simulink model "c_station_v3"  (R2019a)
settings: Solver=VariableStepAuto  StartTime=0.0  StopTime=604800  MaxStep=3600  RelTol=1e-3  AbsTol=1e-3  EnableMultiTasking=on
StopFcn:
  | displayGasParameters(gasPressures);
values from neighbouring files (symbols this model uses):
  conf = gasConfig()    [gas_v1.m]
  valveControlFlag = "on"    [gas_v1.m]
undefined symbols (not defined in the file or in its folder): lineParm, loadParm, valveParm
libraries: gasLibrary x25, fl_lib x19, nesl_utility x11, SimscapeFluids_lib x1
(part 3 of 3)

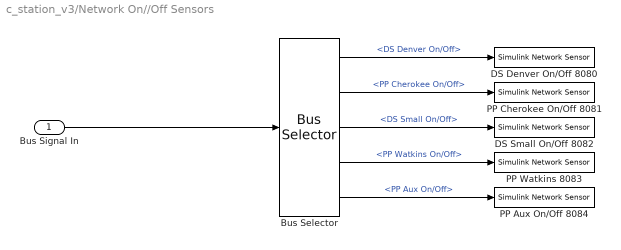
== system c_station_v3/Network On//Off Sensors ==
  Bus Signal In : Inport
  Bus Selector : BusSelector  OutputSignals=DS Denver On/Off,PP Cherokee On/Off,DS Small On/Off,PP Watkins On/Off,PP Aux On/Off
  DS Denver On/Off 8080 : gasLibrary/Simulink Network Sensor  Port=8080
  DS Small On/Off 8082 : gasLibrary/Simulink Network Sensor  Port=8082
  PP Aux On/Off 8084 : gasLibrary/Simulink Network Sensor  Port=8084
  PP Cherokee On/Off 8081 : gasLibrary/Simulink Network Sensor  Port=8081
  PP Watkins 8083 : gasLibrary/Simulink Network Sensor  Port=8083
  wires:
  Bus Selector/1 -> DS Denver On/Off 8080/1  "<DS Denver On/Off>"
  Bus Signal In/1 -> Bus Selector/1
  Bus Selector/2 -> PP Cherokee On/Off 8081/1  "<PP Cherokee On/Off>"
  Bus Selector/4 -> PP Watkins 8083/1  "<PP Watkins On/Off>"
  Bus Selector/5 -> PP Aux On/Off 8084/1  "<PP Aux On/Off>"
  Bus Selector/3 -> DS Small On/Off 8082/1  "<DS Small On/Off>"

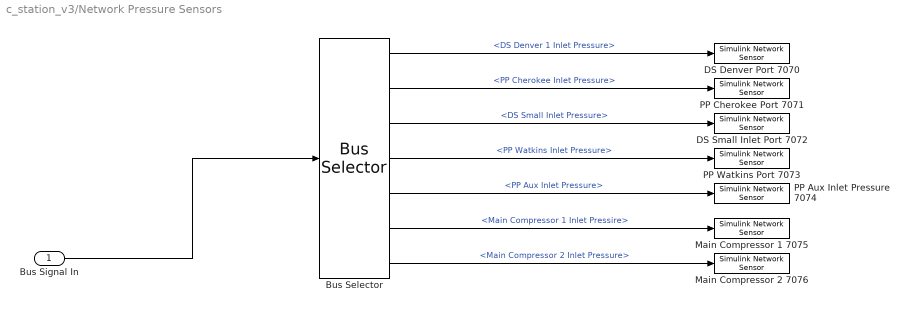
== system c_station_v3/Network Pressure Sensors ==
  Bus Signal In : Inport
  Bus Selector : BusSelector  OutputSignals=DS Denver 1 Inlet Pressure,PP Cherokee Inlet Pressure,DS Small Inlet Pressure,PP Watkins Inlet Pressure,PP Aux Inlet Pressure,Main Compressor 1 Inlet Pressire,Main Compressor 2 Inlet Pressure
  DS Denver Port 7070 : gasLibrary/Simulink Network Sensor  Port=7070
  DS Small Inlet Port 7072 : gasLibrary/Simulink Network Sensor  Port=7072
  Main Compressor 1 7075 : gasLibrary/Simulink Network Sensor  Port=7075
  Main Compressor 2 7076 : gasLibrary/Simulink Network Sensor  Port=7076
  PP Aux Inlet Pressure 7074 : gasLibrary/Simulink Network Sensor  Port=7074
  PP Cherokee Port 7071 : gasLibrary/Simulink Network Sensor  Port=7071
  PP Watkins Port 7073 : gasLibrary/Simulink Network Sensor  Port=7073
  wires:
  Bus Selector/4 -> PP Watkins Port 7073/1  "<PP Watkins Inlet Pressure>"
  Bus Signal In/1 -> Bus Selector/1
  Bus Selector/2 -> PP Cherokee Port 7071/1  "<PP Cherokee Inlet Pressure>"
  Bus Selector/3 -> DS Small Inlet Port 7072/1  "<DS Small Inlet Pressure>"
  Bus Selector/1 -> DS Denver Port 7070/1  "<DS Denver 1 Inlet Pressure>"
  Bus Selector/6 -> Main Compressor 1 7075/1  "<Main Compressor 1 Inlet Pressire>"
  Bus Selector/7 -> Main Compressor 2 7076/1  "<Main Compressor 2 Inlet Pressure>"
  Bus Selector/5 -> PP Aux Inlet Pressure 7074/1  "<PP Aux Inlet Pressure>"

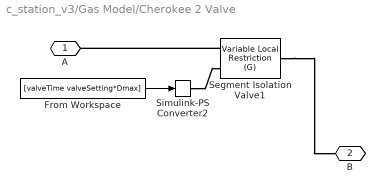
== system c_station_v3/Gas Model/Cherokee 2 Valve ==
  From Workspace : FromWorkspace  VariableName=[valveTime valveSetting*Dmax]  SampleTime=0  OutputAfterFinalValue=Holding final value
  Segment Isolation Valve1 : fl_lib/Gas/Elements/Variable Local Restriction (G)  min_area=1e-4 in^2  max_area=pi*(Dmax-1)^2/4 in^2  area=pi*D^2/4 in^2  Cd=0.64  B_lam=0.999  mdot_A_specify=off  mdot_A_priority=None  mdot_A=1e-6 kg/s  mdot_A_nominal_specify=off  mdot_A_nominal_unit=kg/s  mdot_A_nominal_value=1
      settings: SourceProductName=Simscape  SourceProductBaseCode=SS
  Simulink-PS Converter2 : nesl_utility/Simulink-PS Converter  PhysicalDomain=network_engine_domain  SubClassName=ps_input  LeftPortType=input  RightPortType=output  PseudoPeriodic=off  Frequencies=[]  NoiseDistribution=none  NoiseParameters=[]  Unit=in^2  AffineConversion=off  FilteringAndDerivatives=provide  SimscapeFilterOrder=1  InputFilterTimeConstant=0.001  UdotUserProvided=0
  A : PMIOPort  Side=Left
  B : PMIOPort  Port=2  Side=Right
  wires:
  From Workspace/1 -> Simulink-PS Converter2/1
  connections:
  Simulink-PS Converter2/RConn1 -- Segment Isolation Valve1/LConn2
  Segment Isolation Valve1/LConn1 -- A/RConn1
  Segment Isolation Valve1/RConn1 -- B/RConn1

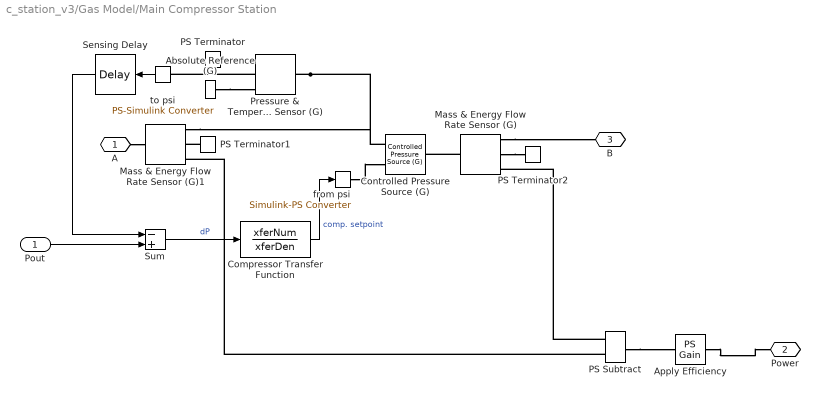
== system c_station_v3/Gas Model/Main Compressor Station ==
  Pout : Inport
  Absolute Reference (G) : fl_lib/Gas/Elements/Absolute Reference (G)
      settings: SourceProductName=Simscape  SourceProductBaseCode=SS
  Apply Efficiency : fl_lib/Physical Signals/Functions/PS Gain  gain=1/efficiency
  Compressor Transfer Function : TransferFcn  Numerator=xferNum  Denominator=xferDen
  Controlled Pressure Source (G) : fl_lib/Gas/Sources/Controlled Pressure Source (G)  power_spec=1  area_A=24^2*pi/4 in^2  area_B=24^2*pi/4 in^2  mdot_A_specify=off  mdot_A_priority=None  mdot_A=1e-6 kg/s  mdot_A_nominal_specify=off  mdot_A_nominal_unit=kg/s  mdot_A_nominal_value=1
      settings: SourceProductName=Simscape  SourceProductBaseCode=SS
  Mass & Energy Flow Rate Sensor (G) : fl_lib/Gas/Sensors/Mass & Energy Flow Rate Sensor (G)
      settings: SourceProductName=Simscape  SourceProductBaseCode=SS
  Mass & Energy Flow Rate Sensor (G)1 : fl_lib/Gas/Sensors/Mass & Energy Flow Rate Sensor (G)
      settings: SourceProductName=Simscape  SourceProductBaseCode=SS
  PS Subtract : fl_lib/Physical Signals/Functions/PS Subtract
      settings: SourceProductName=Simscape
  PS Terminator : fl_lib/Physical Signals/Sinks/PS Terminator
      settings: SourceProductName=Simscape
  PS Terminator1 : fl_lib/Physical Signals/Sinks/PS Terminator
      settings: SourceProductName=Simscape
  PS Terminator2 : fl_lib/Physical Signals/Sinks/PS Terminator
      settings: SourceProductName=Simscape
  Pressure & Temperature Sensor (G) : fl_lib/Gas/Sensors/Pressure & Temperature Sensor (G)
      settings: SourceProductName=Simscape  SourceProductBaseCode=SS
  Sensing Delay : TransportDelay  DelayTime=delaySeconds  TransDelayFeedthrough=on
  Sum : Sum  Inputs=-+
  from psi : nesl_utility/Simulink-PS Converter  PhysicalDomain=network_engine_domain  SubClassName=ps_input  LeftPortType=input  RightPortType=output  PseudoPeriodic=off  Frequencies=[]  NoiseDistribution=none  NoiseParameters=[]  Unit=psi  AffineConversion=off  FilteringAndDerivatives=provide  SimscapeFilterOrder=1  InputFilterTimeConstant=0.001  UdotUserProvided=0
  to psi : nesl_utility/PS-Simulink Converter  PhysicalDomain=network_engine_domain  SubClassName=ps_output  LeftPortType=input  RightPortType=output  PseudoPeriodic=off  Frequencies=[]  Unit=psi  AffineConversion=off
  A : PMIOPort  Side=Left
  Power : PMIOPort  Port=2  Side=Right
  B : PMIOPort  Port=3  Side=Right
  wires:
  to psi/1 -> Sensing Delay/1
  Sensing Delay/1 -> Sum/1
  Compressor Transfer Function/1 -> from psi/1  "comp. setpoint"
  Sum/1 -> Compressor Transfer Function/1  "dP"
  Pout/1 -> Sum/2
  connections:
  Apply Efficiency/RConn1 -- Power/RConn1
  PS Subtract/RConn1 -- Apply Efficiency/LConn1
  PS Subtract/LConn2 -- Mass & Energy Flow Rate Sensor (G)1/RConn3
  PS Subtract/LConn1 -- Mass & Energy Flow Rate Sensor (G)/RConn3
  Mass & Energy Flow Rate Sensor (G)/RConn2 -- PS Terminator2/LConn1
  PS Terminator1/LConn1 -- Mass & Energy Flow Rate Sensor (G)1/RConn2
  A/RConn1 -- Mass & Energy Flow Rate Sensor (G)1/LConn1
  Mass & Energy Flow Rate Sensor (G)/RConn1 -- B/RConn1
  Mass & Energy Flow Rate Sensor (G)/LConn1 -- Controlled Pressure Source (G)/RConn1
  Pressure & Temperature Sensor (G)/LConn1 -- Mass & Energy Flow Rate Sensor (G)1/RConn1 -- Controlled Pressure Source (G)/LConn1
  PS Terminator/LConn1 -- Pressure & Temperature Sensor (G)/RConn3
  from psi/RConn1 -- Controlled Pressure Source (G)/LConn2
  Pressure & Temperature Sensor (G)/RConn2 -- to psi/LConn1
  Absolute Reference (G)/LConn1 -- Pressure & Temperature Sensor (G)/RConn1

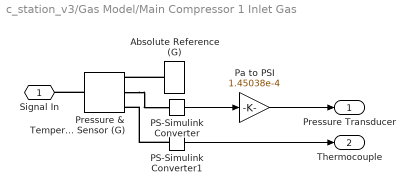
== system c_station_v3/Gas Model/Main Compressor 1 Inlet Gas ==
  Absolute Reference (G) : fl_lib/Gas/Elements/Absolute Reference (G)
      settings: SourceProductName=Simscape  SourceProductBaseCode=SS
  PS-Simulink Converter : nesl_utility/PS-Simulink Converter  PhysicalDomain=network_engine_domain  SubClassName=ps_output  LeftPortType=input  RightPortType=output  PseudoPeriodic=off  Frequencies=[]  Unit=1  AffineConversion=off
  PS-Simulink Converter1 : nesl_utility/PS-Simulink Converter  PhysicalDomain=network_engine_domain  SubClassName=ps_output  LeftPortType=input  RightPortType=output  PseudoPeriodic=off  Frequencies=[]  Unit=1  AffineConversion=off
  Pa to PSI : Gain  Gain=1.45038e-4
  Pressure & Temperature Sensor (G) : fl_lib/Gas/Sensors/Pressure & Temperature Sensor (G)
      settings: SourceProductName=Simscape  SourceProductBaseCode=SS
  Signal In : PMIOPort  Side=Left
  Pressure Transducer : Outport
  Thermocouple : Outport  Port=2
  wires:
  PS-Simulink Converter/1 -> Pa to PSI/1
  PS-Simulink Converter1/1 -> Thermocouple/1
  Pa to PSI/1 -> Pressure Transducer/1
  connections:
  Pressure & Temperature Sensor (G)/LConn1 -- Signal In/RConn1
  Absolute Reference (G)/LConn1 -- Pressure & Temperature Sensor (G)/RConn1
  PS-Simulink Converter1/LConn1 -- Pressure & Temperature Sensor (G)/RConn3
  Pressure & Temperature Sensor (G)/RConn2 -- PS-Simulink Converter/LConn1

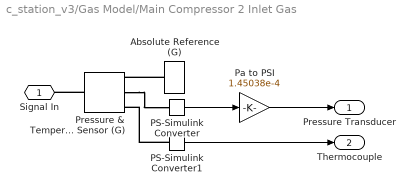
== system c_station_v3/Gas Model/Main Compressor 2 Inlet Gas ==
  Absolute Reference (G) : fl_lib/Gas/Elements/Absolute Reference (G)
      settings: SourceProductName=Simscape  SourceProductBaseCode=SS
  PS-Simulink Converter : nesl_utility/PS-Simulink Converter  PhysicalDomain=network_engine_domain  SubClassName=ps_output  LeftPortType=input  RightPortType=output  PseudoPeriodic=off  Frequencies=[]  Unit=1  AffineConversion=off
  PS-Simulink Converter1 : nesl_utility/PS-Simulink Converter  PhysicalDomain=network_engine_domain  SubClassName=ps_output  LeftPortType=input  RightPortType=output  PseudoPeriodic=off  Frequencies=[]  Unit=1  AffineConversion=off
  Pa to PSI : Gain  Gain=1.45038e-4
  Pressure & Temperature Sensor (G) : fl_lib/Gas/Sensors/Pressure & Temperature Sensor (G)
      settings: SourceProductName=Simscape  SourceProductBaseCode=SS
  Signal In : PMIOPort  Side=Left
  Pressure Transducer : Outport
  Thermocouple : Outport  Port=2
  wires:
  PS-Simulink Converter/1 -> Pa to PSI/1
  PS-Simulink Converter1/1 -> Thermocouple/1
  Pa to PSI/1 -> Pressure Transducer/1
  connections:
  Pressure & Temperature Sensor (G)/LConn1 -- Signal In/RConn1
  Absolute Reference (G)/LConn1 -- Pressure & Temperature Sensor (G)/RConn1
  PS-Simulink Converter1/LConn1 -- Pressure & Temperature Sensor (G)/RConn3
  Pressure & Temperature Sensor (G)/RConn2 -- PS-Simulink Converter/LConn1

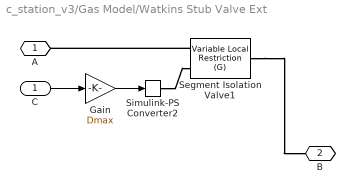
== system c_station_v3/Gas Model/Watkins Stub Valve Ext ==
  C : Inport
  Gain : Gain  Gain=Dmax
  Segment Isolation Valve1 : fl_lib/Gas/Elements/Variable Local Restriction (G)  min_area=1e-4 in^2  max_area=pi*(Dmax-1)^2/4 in^2  area=pi*D^2/4 in^2  Cd=0.64  B_lam=0.999  mdot_A_specify=off  mdot_A_priority=None  mdot_A=1e-6 kg/s  mdot_A_nominal_specify=off  mdot_A_nominal_unit=kg/s  mdot_A_nominal_value=1
      settings: SourceProductName=Simscape  SourceProductBaseCode=SS
  Simulink-PS Converter2 : nesl_utility/Simulink-PS Converter  PhysicalDomain=network_engine_domain  SubClassName=ps_input  LeftPortType=input  RightPortType=output  PseudoPeriodic=off  Frequencies=[]  NoiseDistribution=none  NoiseParameters=[]  Unit=in^2  AffineConversion=off  FilteringAndDerivatives=provide  SimscapeFilterOrder=1  InputFilterTimeConstant=0.001  UdotUserProvided=0
  A : PMIOPort  Side=Left
  B : PMIOPort  Port=2  Side=Right
  wires:
  C/1 -> Gain/1
  Gain/1 -> Simulink-PS Converter2/1
  connections:
  Segment Isolation Valve1/RConn1 -- B/RConn1
  Segment Isolation Valve1/LConn1 -- A/RConn1
  Simulink-PS Converter2/RConn1 -- Segment Isolation Valve1/LConn2
